simulink model "Arduino_Temp_Model"  (R2016a)
settings: Solver=FixedStepAuto  StartTime=0.0  StopTime=inf  RelTol=1e-3
libraries: arduinolib x1, simulink_extras x1
settings Model: SimulationMode=external  ExtModeTrigDuration=2  Creator=Lara  LastModifiedBy=Lara
settings OptimizationCC: OptimizeModelRefInitCode=on  LifeSpan=1  MaxStackSize=64
settings HardwareCC: ProdBitPerInt=16  ProdBitPerPointer=16  ProdLargestAtomicFloat=None  ProdWordSize=8  ProdHWDeviceType=Atmel->AVR  UseEmbeddedCoderFeatures=off  UseSimulinkCoderFeatures=off
settings RTWCC: SystemTargetFile=ert.tlc  HardwareBoard=Arduino Uno  TemplateMakefile=ert_default_tmf  RTWVerbose=off  Toolchain=Arduino AVR v1.6.1  BuildConfiguration=Faster Runs  IncludeHyperlinkInReport=on
settings CodeAppCC: ForceParamTrailComments=on  OperatorAnnotations=on  SimulinkDataObjDesc=on  SFDataObjDesc=on  MATLABFcnDesc=on  MangleLength=10  InsertBlockDesc=on  MATLABSourceComments=on
settings ERTTargetCC: SupportContinuousTime=on  SupportNonInlinedSFcns=on  SupportVariableSizeSignals=on  ExtMode=on  ExtModeTransport=3  ExtModeMexFile=ext_serial_win32_comm_rtt  ExtModeMexArgs=0 4 115200  ERTSrcFileBannerTemplate=codertarget_code_template.cgt  ERTHdrFileBannerTemplate=codertarget_code_template.cgt  ERTDataSrcFileTemplate=codertarget_code_template.cgt  ERTDataHdrFileTemplate=codertarget_code_template.cgt

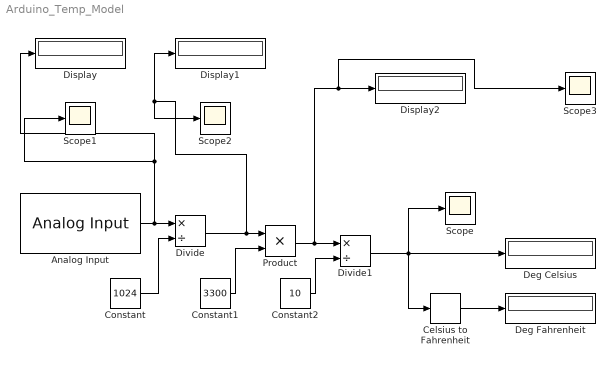
== system Arduino_Temp_Model ==
  Analog Input : arduinolib/Analog Input  pinNumber=1  sampleTime=0.01  blockPlatform=arduino
  Celsius to Fahrenheit : simulink_extras/Transformations/Celsius to Fahrenheit
  Constant : Constant  Value=1024
  Constant1 : Constant  Value=3300
  Constant2 : Constant  Value=10
  Deg Celsius : Display
  Deg Fahrenheit : Display
  Display : Display
  Display1 : Display
  Display2 : Display
  Divide : Product  Inputs=*/
  Divide1 : Product  Inputs=*/
  Product : Product
  Scope{,1..3} (4 alike) : Scope
  wires:
  Celsius to Fahrenheit/1 -> Deg Fahrenheit/1
  Divide1/1 -> Celsius to Fahrenheit/1, Deg Celsius/1, Scope/1
  Constant2/1 -> Divide1/2
  Product/1 -> Scope3/1, Display2/1, Divide1/1
  Constant1/1 -> Product/2
  Divide/1 -> Display1/1, Scope2/1, Product/1
  Constant/1 -> Divide/2
  Analog Input/1 -> Display/1, Scope1/1, Divide/1
